simulink model "HIL_Testing_SW"  (Simulink 7.5)
settings: Solver=ode1  StartTime=0.0  StopTime=Inf  FixedStep=0.001  RelTol=1e-3
PostLoadFcn:
  | , if any(exist('dsrtsu_mdlpostloadfcn', 'file') == [2, 3, 6]), try dsrtsu_mdlpostloadfcn('Execute', bdroot); catch fprintf('Error in PostLoadFcn (dsrtsu_mdlpostloadfcn) for model "%s":\n %s\n', bdroot, lasterr); end, end,
undefined symbols (not defined in the file): CeBSER_Cnt_NumTempAxisPts, ChargeCord, ChargeCord_Control, ChargeToSOCCurr, ChrgCurrLim, CrntSens1Fine, CS_SOCSetPt, CyclerMaxChrgPwr, CyclerMaxDschrgPwr, deltaAhr, Drive_1, Drive_10, Drive_11, Drive_12, Drive_13, Drive_14, Drive_15, Drive_16, Drive_17, Drive_18, Drive_19, Drive_2, Drive_20, Drive_21, Drive_22, Drive_23, Drive_24, Drive_25, Drive_26, Drive_27, Drive_28, Drive_29, Drive_3, Drive_30, Drive_31, Drive_32, Drive_33, Drive_34, Drive_35, Drive_36, Drive_37, Drive_38, Drive_39, Drive_4, Drive_40, Drive_41, Drive_42, Drive_43, Drive_44, Drive_45, Drive_46, Drive_47, Drive_48, Drive_49, Drive_5, Drive_50, Drive_51, Drive_6, Drive_7, Drive_8 ... (+50)
libraries: simulink x129, rtican x50, rti2211sailib x5, rti2211serlib x5, rti2202miolib x3
(part 19 of 23)

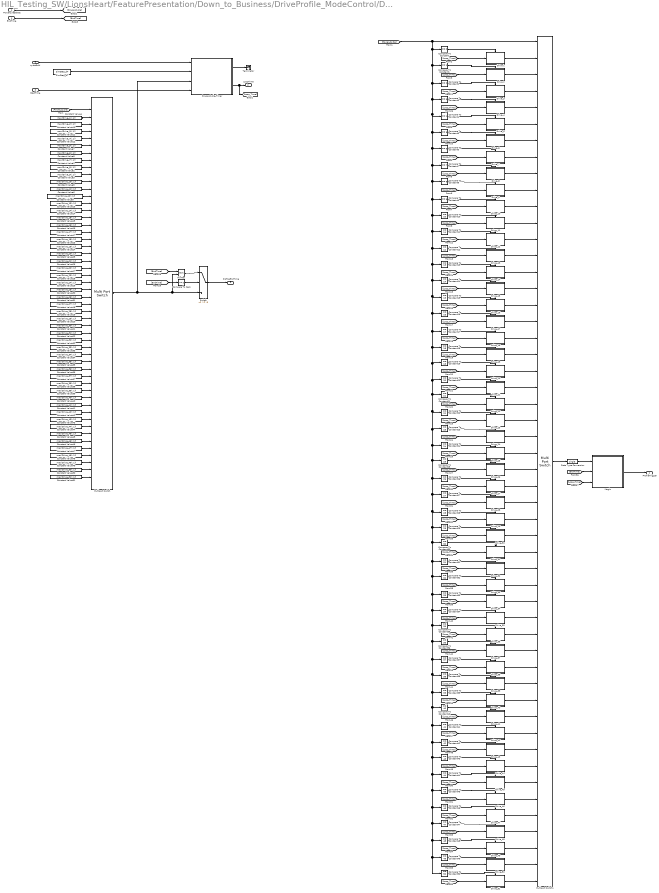
== system HIL_Testing_SW/LionsHeart/FeaturePresentation/Down_to_Business/DriveProfile_ModeControl/Drive_Profile/CD ==
  PowercyleSelect : Inport  OutDataType=fixdt(1, 16)  OutScaling=2^0
  cycleEnbl : Inport  Port=2  OutDataType=fixdt(1, 16)  OutScaling=2^0
  StartTime : Inport  Port=3  OutDataType=fixdt(1, 16)  OutScaling=2^0
  EndTime : Inport  Port=4  OutDataType=fixdt(1, 16)  OutScaling=2^0
  Compare To Constant : simulink/Logic and Bit Operations/Compare To Constant  SystemSampleTime=-1  relop===  const=0  LogicOutDataTypeMode=uint8
  Compare To Constant1 : simulink/Logic and Bit Operations/Compare To Constant  SystemSampleTime=-1  relop===  const=1  LogicOutDataTypeMode=uint8
  Compare To Constant10 : simulink/Logic and Bit Operations/Compare To Constant  SystemSampleTime=-1  relop===  const=10  LogicOutDataTypeMode=uint8
  Compare To Constant11 : simulink/Logic and Bit Operations/Compare To Constant  SystemSampleTime=-1  relop===  const=11  LogicOutDataTypeMode=uint8
  Compare To Constant12 : simulink/Logic and Bit Operations/Compare To Constant  SystemSampleTime=-1  relop===  const=12  LogicOutDataTypeMode=uint8
  Compare To Constant13 : simulink/Logic and Bit Operations/Compare To Constant  SystemSampleTime=-1  relop===  const=13  LogicOutDataTypeMode=uint8
  Compare To Constant14 : simulink/Logic and Bit Operations/Compare To Constant  SystemSampleTime=-1  relop===  const=14  LogicOutDataTypeMode=uint8
  Compare To Constant15 : simulink/Logic and Bit Operations/Compare To Constant  SystemSampleTime=-1  relop===  const=15  LogicOutDataTypeMode=uint8
  Compare To Constant16 : simulink/Logic and Bit Operations/Compare To Constant  SystemSampleTime=-1  relop===  const=16  LogicOutDataTypeMode=uint8
  Compare To Constant17 : simulink/Logic and Bit Operations/Compare To Constant  SystemSampleTime=-1  relop===  const=17  LogicOutDataTypeMode=uint8
  Compare To Constant18 : simulink/Logic and Bit Operations/Compare To Constant  SystemSampleTime=-1  relop===  const=18  LogicOutDataTypeMode=uint8
  Compare To Constant19 : simulink/Logic and Bit Operations/Compare To Constant  SystemSampleTime=-1  relop===  const=19  LogicOutDataTypeMode=uint8
  Compare To Constant2 : simulink/Logic and Bit Operations/Compare To Constant  SystemSampleTime=-1  relop===  const=2  LogicOutDataTypeMode=uint8
  Compare To Constant20 : simulink/Logic and Bit Operations/Compare To Constant  SystemSampleTime=-1  relop===  const=20  LogicOutDataTypeMode=uint8
  Compare To Constant21 : simulink/Logic and Bit Operations/Compare To Constant  SystemSampleTime=-1  relop===  const=21  LogicOutDataTypeMode=uint8
  Compare To Constant22 : simulink/Logic and Bit Operations/Compare To Constant  SystemSampleTime=-1  relop===  const=22  LogicOutDataTypeMode=uint8
  Compare To Constant23 : simulink/Logic and Bit Operations/Compare To Constant  SystemSampleTime=-1  relop===  const=23  LogicOutDataTypeMode=uint8
  Compare To Constant24 : simulink/Logic and Bit Operations/Compare To Constant  SystemSampleTime=-1  relop===  const=24  LogicOutDataTypeMode=uint8
  Compare To Constant25 : simulink/Logic and Bit Operations/Compare To Constant  SystemSampleTime=-1  relop===  const=25  LogicOutDataTypeMode=uint8
  Compare To Constant26 : simulink/Logic and Bit Operations/Compare To Constant  SystemSampleTime=-1  relop===  const=26  LogicOutDataTypeMode=uint8
  Compare To Constant27 : simulink/Logic and Bit Operations/Compare To Constant  SystemSampleTime=-1  relop===  const=27  LogicOutDataTypeMode=uint8
  Compare To Constant28 : simulink/Logic and Bit Operations/Compare To Constant  SystemSampleTime=-1  relop===  const=28  LogicOutDataTypeMode=uint8
  Compare To Constant29 : simulink/Logic and Bit Operations/Compare To Constant  SystemSampleTime=-1  relop===  const=29  LogicOutDataTypeMode=uint8
  Compare To Constant3 : simulink/Logic and Bit Operations/Compare To Constant  SystemSampleTime=-1  relop===  const=3  LogicOutDataTypeMode=uint8
  Compare To Constant30 : simulink/Logic and Bit Operations/Compare To Constant  SystemSampleTime=-1  relop===  const=30  LogicOutDataTypeMode=uint8
  Compare To Constant31 : simulink/Logic and Bit Operations/Compare To Constant  SystemSampleTime=-1  relop===  const=31  LogicOutDataTypeMode=uint8
  Compare To Constant32 : simulink/Logic and Bit Operations/Compare To Constant  SystemSampleTime=-1  relop===  const=32  LogicOutDataTypeMode=uint8
  Compare To Constant33 : simulink/Logic and Bit Operations/Compare To Constant  SystemSampleTime=-1  relop===  const=33  LogicOutDataTypeMode=uint8
  Compare To Constant34 : simulink/Logic and Bit Operations/Compare To Constant  SystemSampleTime=-1  relop===  const=34  LogicOutDataTypeMode=uint8
  Compare To Constant35 : simulink/Logic and Bit Operations/Compare To Constant  SystemSampleTime=-1  relop===  const=35  LogicOutDataTypeMode=uint8
  Compare To Constant36 : simulink/Logic and Bit Operations/Compare To Constant  SystemSampleTime=-1  relop===  const=36  LogicOutDataTypeMode=uint8
  Compare To Constant37 : simulink/Logic and Bit Operations/Compare To Constant  SystemSampleTime=-1  relop===  const=37  LogicOutDataTypeMode=uint8
  Compare To Constant38 : simulink/Logic and Bit Operations/Compare To Constant  SystemSampleTime=-1  relop===  const=38  LogicOutDataTypeMode=uint8
  Compare To Constant39 : simulink/Logic and Bit Operations/Compare To Constant  SystemSampleTime=-1  relop===  const=39  LogicOutDataTypeMode=uint8
  Compare To Constant4 : simulink/Logic and Bit Operations/Compare To Constant  SystemSampleTime=-1  relop===  const=4  LogicOutDataTypeMode=uint8
  Compare To Constant40 : simulink/Logic and Bit Operations/Compare To Constant  SystemSampleTime=-1  relop===  const=40  LogicOutDataTypeMode=uint8
  Compare To Constant41 : simulink/Logic and Bit Operations/Compare To Constant  SystemSampleTime=-1  relop===  const=41  LogicOutDataTypeMode=uint8
  Compare To Constant42 : simulink/Logic and Bit Operations/Compare To Constant  SystemSampleTime=-1  relop===  const=42  LogicOutDataTypeMode=uint8
  Compare To Constant43 : simulink/Logic and Bit Operations/Compare To Constant  SystemSampleTime=-1  relop===  const=43  LogicOutDataTypeMode=uint8
  Compare To Constant44 : simulink/Logic and Bit Operations/Compare To Constant  SystemSampleTime=-1  relop===  const=44  LogicOutDataTypeMode=uint8
  Compare To Constant45 : simulink/Logic and Bit Operations/Compare To Constant  SystemSampleTime=-1  relop===  const=45  LogicOutDataTypeMode=uint8
  Compare To Constant46 : simulink/Logic and Bit Operations/Compare To Constant  SystemSampleTime=-1  relop===  const=46  LogicOutDataTypeMode=uint8
  Compare To Constant47 : simulink/Logic and Bit Operations/Compare To Constant  SystemSampleTime=-1  relop===  const=47  LogicOutDataTypeMode=uint8
  Compare To Constant48 : simulink/Logic and Bit Operations/Compare To Constant  SystemSampleTime=-1  relop===  const=48  LogicOutDataTypeMode=uint8
  Compare To Constant49 : simulink/Logic and Bit Operations/Compare To Constant  SystemSampleTime=-1  relop===  const=49  LogicOutDataTypeMode=uint8
  Compare To Constant5 : simulink/Logic and Bit Operations/Compare To Constant  SystemSampleTime=-1  relop===  const=5  LogicOutDataTypeMode=uint8
  Compare To Constant50 : simulink/Logic and Bit Operations/Compare To Constant  SystemSampleTime=-1  relop===  const=50  LogicOutDataTypeMode=uint8
  Compare To Constant6 : simulink/Logic and Bit Operations/Compare To Constant  SystemSampleTime=-1  relop===  const=6  LogicOutDataTypeMode=uint8
  Compare To Constant7 : simulink/Logic and Bit Operations/Compare To Constant  SystemSampleTime=-1  relop===  const=7  LogicOutDataTypeMode=uint8
  Compare To Constant8 : simulink/Logic and Bit Operations/Compare To Constant  SystemSampleTime=-1  relop===  const=8  LogicOutDataTypeMode=uint8
  Compare To Constant9 : simulink/Logic and Bit Operations/Compare To Constant  SystemSampleTime=-1  relop===  const=9  LogicOutDataTypeMode=uint8
  Compare To Zero : simulink/Logic and Bit Operations/Compare To Zero  SystemSampleTime=-1  relop=~=  LogicOutDataTypeMode=boolean
  Constant Value1 : Constant  Tag=R12-1  Value=max(Drive_7(:,1))  OutDataType=sfix(16)  OutScaling=2^0
  Constant Value10 : Constant  Tag=R12-1  Value=max(Drive_2(:,1))  OutDataType=sfix(16)  OutScaling=2^0
  Constant Value11 : Constant  Tag=R12-1  Value=max(Drive_3(:,1))  OutDataType=sfix(16)  OutScaling=2^0
  Constant Value12 : Constant  Tag=R12-1  Value=max(Drive_4(:,1))  OutDataType=sfix(16)  OutScaling=2^0
  Constant Value13 : Constant  Tag=R12-1  Value=max(Drive_13(:,1))  OutDataType=sfix(16)  OutScaling=2^0
  Constant Value14 : Constant  Tag=R12-1  Value=max(Drive_14(:,1))  OutDataType=sfix(16)  OutScaling=2^0
  Constant Value15 : Constant  Tag=R12-1  Value=max(Drive_15(:,1))  OutDataType=sfix(16)  OutScaling=2^0
  Constant Value16 : Constant  Tag=R12-1  Value=max(Drive_16(:,1))  OutDataType=sfix(16)  OutScaling=2^0
  Constant Value17 : Constant  Tag=R12-1  Value=max(Drive_17(:,1))  OutDataType=sfix(16)  OutScaling=2^0
  Constant Value18 : Constant  Tag=R12-1  Value=max(Drive_27(:,1))  OutDataType=sfix(16)  OutScaling=2^0
  Constant Value19 : Constant  Tag=R12-1  Value=max(Drive_28(:,1))  OutDataType=sfix(16)  OutScaling=2^0
  Constant Value2 : Constant  Tag=R12-1  Value=max(Drive_8(:,1))  OutDataType=sfix(16)  OutScaling=2^0
  Constant Value20 : Constant  Tag=R12-1  Value=max(Drive_29(:,1))  OutDataType=sfix(16)  OutScaling=2^0
  Constant Value21 : Constant  Tag=R12-1  Value=max(Drive_30(:,1))  OutDataType=sfix(16)  OutScaling=2^0
  Constant Value22 : Constant  Tag=R12-1  Value=max(Drive_31(:,1))  OutDataType=sfix(16)  OutScaling=2^0
  Constant Value23 : Constant  Tag=R12-1  Value=max(Drive_18(:,1))  OutDataType=sfix(16)  OutScaling=2^0
  Constant Value24 : Constant  Tag=R12-1  Value=max(Drive_19(:,1))  OutDataType=sfix(16)  OutScaling=2^0
  Constant Value25 : Constant  Tag=R12-1  Value=max(Drive_20(:,1))  OutDataType=sfix(16)  OutScaling=2^0
  Constant Value26 : Constant  Tag=R12-1  Value=max(Drive_21(:,1))  OutDataType=sfix(16)  OutScaling=2^0
  Constant Value27 : Constant  Tag=R12-1  Value=max(Drive_22(:,1))  OutDataType=sfix(16)  OutScaling=2^0
  Constant Value28 : Constant  Tag=R12-1  Value=max(Drive_23(:,1))  VectorParams1D=off  OutDataType=sfix(16)  OutScaling=2^0
  Constant Value29 : Constant  Tag=R12-1  Value=max(Drive_24(:,1))  OutDataType=sfix(16)  OutScaling=2^0
  Constant Value3 : Constant  Tag=R12-1  Value=max(Drive_9(:,1))  OutDataType=sfix(16)  OutScaling=2^0
  Constant Value30 : Constant  Tag=R12-1  Value=max(Drive_25(:,1))  OutDataType=sfix(16)  OutScaling=2^0
  Constant Value31 : Constant  Tag=R12-1  Value=max(Drive_26(:,1))  OutDataType=sfix(16)  OutScaling=2^0
  Constant Value32 : Constant  Tag=R12-1  Value=max(Drive_32(:,1))  OutDataType=sfix(16)  OutScaling=2^0
  Constant Value33 : Constant  Tag=R12-1  Value=max(Drive_33(:,1))  OutDataType=sfix(16)  OutScaling=2^0
  Constant Value34 : Constant  Tag=R12-1  Value=max(Drive_34(:,1))  OutDataType=sfix(16)  OutScaling=2^0
  Constant Value35 : Constant  Tag=R12-1  Value=max(Drive_35(:,1))  OutDataType=sfix(16)  OutScaling=2^0
  Constant Value36 : Constant  Tag=R12-1  Value=max(Drive_36(:,1))  OutDataType=sfix(16)  OutScaling=2^0
  Constant Value37 : Constant  Tag=R12-1  Value=max(Drive_37(:,1))  OutDataType=sfix(16)  OutScaling=2^0
  Constant Value38 : Constant  Tag=R12-1  Value=max(Drive_38(:,1))  OutDataType=sfix(16)  OutScaling=2^0
  Constant Value39 : Constant  Tag=R12-1  Value=max(Drive_39(:,1))  OutDataType=sfix(16)  OutScaling=2^0
  Constant Value4 : Constant  Tag=R12-1  Value=max(Drive_1(:,1))  OutDataType=sfix(16)  OutScaling=2^0
  Constant Value40 : Constant  Tag=R12-1  Value=max(Drive_40(:,1))  OutDataType=sfix(16)  OutScaling=2^0
  Constant Value41 : Constant  Tag=R12-1  Value=max(Drive_41(:,1))  OutDataType=sfix(16)  OutScaling=2^0
  Constant Value42 : Constant  Tag=R12-1  Value=max(Drive_42(:,1))  OutDataType=sfix(16)  OutScaling=2^0
  Constant Value43 : Constant  Tag=R12-1  Value=max(Drive_43(:,1))  OutDataType=sfix(16)  OutScaling=2^0
  Constant Value44 : Constant  Tag=R12-1  Value=max(Drive_44(:,1))  OutDataType=sfix(16)  OutScaling=2^0
  Constant Value45 : Constant  Tag=R12-1  Value=max(Drive_45(:,1))  OutDataType=sfix(16)  OutScaling=2^0
  Constant Value46 : Constant  Tag=R12-1  Value=max(Drive_46(:,1))  OutDataType=sfix(16)  OutScaling=2^0
  Constant Value47 : Constant  Tag=R12-1  Value=max(Drive_47(:,1))  OutDataType=sfix(16)  OutScaling=2^0
  Constant Value48 : Constant  Tag=R12-1  Value=max(Drive_48(:,1))  OutDataType=sfix(16)  OutScaling=2^0
  Constant Value49 : Constant  Tag=R12-1  Value=max(Drive_49(:,1))  OutDataType=sfix(16)  OutScaling=2^0
  Constant Value5 : Constant  Tag=R12-1  Value=max(Drive_10(:,1))  OutDataType=sfix(16)  OutScaling=2^0
  Constant Value50 : Constant  Tag=R12-1  Value=max(Drive_50(:,1))  OutDataType=sfix(16)  OutScaling=2^0
  Constant Value51 : Constant  Tag=R12-1  Value=max(Drive_51(:,1))  OutDataType=sfix(16)  OutScaling=2^0
  Constant Value6 : Constant  Tag=R12-1  Value=max(Drive_11(:,1))  OutDataType=sfix(16)  OutScaling=2^0
  Constant Value7 : Constant  Tag=R12-1  Value=max(Drive_5(:,1))  OutDataType=sfix(16)  OutScaling=2^0
  Constant Value8 : Constant  Tag=R12-1  Value=max(Drive_6(:,1))  VectorParams1D=off  OutDataType=sfix(16)  OutScaling=2^0
  Constant Value9 : Constant  Tag=R12-1  Value=max(Drive_12(:,1))  OutDataType=sfix(16)  OutScaling=2^0
  Data Type Conversion : DataTypeConversion  OutDataTypeMode=single  OutDataType=sfix(16)  OutScaling=2^0  OutDataTypeStr=single
  Drive 1 : Subsystem  Tag=x.x
      mask Type: Subsystem
      mask Display:
      | text(.52,.01,char(get_param(gcb,'Tag') ), 'horizontalAlignment','center','verticalAlignment','bottom' )
      | disp(get_param(gcb,'Name'))
  Drive 2 : Subsystem  Tag=x.x
      mask Type: Subsystem
      mask Display:
      | text(.52,.01,char(get_param(gcb,'Tag') ), 'horizontalAlignment','center','verticalAlignment','bottom' )
      | disp(get_param(gcb,'Name'))
  Drive_10 : Subsystem  Tag=x.x
      mask Type: Subsystem
      mask Display:
      | text(.52,.01,char(get_param(gcb,'Tag') ), 'horizontalAlignment','center','verticalAlignment','bottom' )
      | disp(get_param(gcb,'Name'))
  Drive_11 : Subsystem  Tag=x.x
      mask Type: Subsystem
      mask Display:
      | text(.52,.01,char(get_param(gcb,'Tag') ), 'horizontalAlignment','center','verticalAlignment','bottom' )
      | disp(get_param(gcb,'Name'))
  Drive_12 : Subsystem  Tag=x.x
      mask Type: Subsystem
      mask Display:
      | text(.52,.01,char(get_param(gcb,'Tag') ), 'horizontalAlignment','center','verticalAlignment','bottom' )
      | disp(get_param(gcb,'Name'))
  Drive_13 : Subsystem  Tag=x.x
      mask Type: Subsystem
      mask Display:
      | text(.52,.01,char(get_param(gcb,'Tag') ), 'horizontalAlignment','center','verticalAlignment','bottom' )
      | disp(get_param(gcb,'Name'))
  Drive_14 : Subsystem  Tag=x.x
      mask Type: Subsystem
      mask Display:
      | text(.52,.01,char(get_param(gcb,'Tag') ), 'horizontalAlignment','center','verticalAlignment','bottom' )
      | disp(get_param(gcb,'Name'))
  Drive_15 : Subsystem  Tag=x.x
      mask Type: Subsystem
      mask Display:
      | text(.52,.01,char(get_param(gcb,'Tag') ), 'horizontalAlignment','center','verticalAlignment','bottom' )
      | disp(get_param(gcb,'Name'))
  Drive_16 : Subsystem  Tag=x.x
      mask Type: Subsystem
      mask Display:
      | text(.52,.01,char(get_param(gcb,'Tag') ), 'horizontalAlignment','center','verticalAlignment','bottom' )
      | disp(get_param(gcb,'Name'))
  Drive_17 : Subsystem  Tag=x.x
      mask Type: Subsystem
      mask Display:
      | text(.52,.01,char(get_param(gcb,'Tag') ), 'horizontalAlignment','center','verticalAlignment','bottom' )
      | disp(get_param(gcb,'Name'))
  Drive_18 : Subsystem  Tag=x.x
      mask Type: Subsystem
      mask Display:
      | text(.52,.01,char(get_param(gcb,'Tag') ), 'horizontalAlignment','center','verticalAlignment','bottom' )
      | disp(get_param(gcb,'Name'))
  Drive_19 : Subsystem  Tag=x.x
      mask Type: Subsystem
      mask Display:
      | text(.52,.01,char(get_param(gcb,'Tag') ), 'horizontalAlignment','center','verticalAlignment','bottom' )
      | disp(get_param(gcb,'Name'))
  Drive_20 : Subsystem  Tag=x.x
      mask Type: Subsystem
      mask Display:
      | text(.52,.01,char(get_param(gcb,'Tag') ), 'horizontalAlignment','center','verticalAlignment','bottom' )
      | disp(get_param(gcb,'Name'))
  Drive_21 : Subsystem  Tag=x.x
      mask Type: Subsystem
      mask Display:
      | text(.52,.01,char(get_param(gcb,'Tag') ), 'horizontalAlignment','center','verticalAlignment','bottom' )
      | disp(get_param(gcb,'Name'))
  Drive_22 : Subsystem  Tag=x.x
      mask Type: Subsystem
      mask Display:
      | text(.52,.01,char(get_param(gcb,'Tag') ), 'horizontalAlignment','center','verticalAlignment','bottom' )
      | disp(get_param(gcb,'Name'))
  Drive_23 : Subsystem  Tag=x.x
      mask Type: Subsystem
      mask Display:
      | text(.52,.01,char(get_param(gcb,'Tag') ), 'horizontalAlignment','center','verticalAlignment','bottom' )
      | disp(get_param(gcb,'Name'))
  Drive_24 : Subsystem  Tag=x.x
      mask Type: Subsystem
      mask Display:
      | text(.52,.01,char(get_param(gcb,'Tag') ), 'horizontalAlignment','center','verticalAlignment','bottom' )
      | disp(get_param(gcb,'Name'))
  Drive_25 : Subsystem  Tag=x.x
      mask Type: Subsystem
      mask Display:
      | text(.52,.01,char(get_param(gcb,'Tag') ), 'horizontalAlignment','center','verticalAlignment','bottom' )
      | disp(get_param(gcb,'Name'))
  Drive_26 : Subsystem  Tag=x.x
      mask Type: Subsystem
      mask Display:
      | text(.52,.01,char(get_param(gcb,'Tag') ), 'horizontalAlignment','center','verticalAlignment','bottom' )
      | disp(get_param(gcb,'Name'))
  Drive_27 : Subsystem  Tag=x.x
      mask Type: Subsystem
      mask Display:
      | text(.52,.01,char(get_param(gcb,'Tag') ), 'horizontalAlignment','center','verticalAlignment','bottom' )
      | disp(get_param(gcb,'Name'))
  Drive_28 : Subsystem  Tag=x.x
      mask Type: Subsystem
      mask Display:
      | text(.52,.01,char(get_param(gcb,'Tag') ), 'horizontalAlignment','center','verticalAlignment','bottom' )
      | disp(get_param(gcb,'Name'))
  Drive_29 : Subsystem  Tag=x.x
      mask Type: Subsystem
      mask Display:
      | text(.52,.01,char(get_param(gcb,'Tag') ), 'horizontalAlignment','center','verticalAlignment','bottom' )
      | disp(get_param(gcb,'Name'))
  Drive_3 : Subsystem  Tag=x.x
      mask Type: Subsystem
      mask Display:
      | text(.52,.01,char(get_param(gcb,'Tag') ), 'horizontalAlignment','center','verticalAlignment','bottom' )
      | disp(get_param(gcb,'Name'))
  Drive_30 : Subsystem  Tag=x.x
      mask Type: Subsystem
      mask Display:
      | text(.52,.01,char(get_param(gcb,'Tag') ), 'horizontalAlignment','center','verticalAlignment','bottom' )
      | disp(get_param(gcb,'Name'))
  Drive_31 : Subsystem  Tag=x.x
      mask Type: Subsystem
      mask Display:
      | text(.52,.01,char(get_param(gcb,'Tag') ), 'horizontalAlignment','center','verticalAlignment','bottom' )
      | disp(get_param(gcb,'Name'))
  Drive_32 : Subsystem  Tag=x.x
      mask Type: Subsystem
      mask Display:
      | text(.52,.01,char(get_param(gcb,'Tag') ), 'horizontalAlignment','center','verticalAlignment','bottom' )
      | disp(get_param(gcb,'Name'))
  Drive_33 : Subsystem  Tag=x.x
      mask Type: Subsystem
      mask Display:
      | text(.52,.01,char(get_param(gcb,'Tag') ), 'horizontalAlignment','center','verticalAlignment','bottom' )
      | disp(get_param(gcb,'Name'))
  Drive_34 : Subsystem  Tag=x.x
      mask Type: Subsystem
      mask Display:
      | text(.52,.01,char(get_param(gcb,'Tag') ), 'horizontalAlignment','center','verticalAlignment','bottom' )
      | disp(get_param(gcb,'Name'))
  Drive_35 : Subsystem  Tag=x.x
      mask Type: Subsystem
      mask Display:
      | text(.52,.01,char(get_param(gcb,'Tag') ), 'horizontalAlignment','center','verticalAlignment','bottom' )
      | disp(get_param(gcb,'Name'))
  Drive_36 : Subsystem  Tag=x.x
      mask Type: Subsystem
      mask Display:
      | text(.52,.01,char(get_param(gcb,'Tag') ), 'horizontalAlignment','center','verticalAlignment','bottom' )
      | disp(get_param(gcb,'Name'))
  Drive_37 : Subsystem  Tag=x.x
      mask Type: Subsystem
      mask Display:
      | text(.52,.01,char(get_param(gcb,'Tag') ), 'horizontalAlignment','center','verticalAlignment','bottom' )
      | disp(get_param(gcb,'Name'))
  Drive_38 : Subsystem  Tag=x.x
      mask Type: Subsystem
      mask Display:
      | text(.52,.01,char(get_param(gcb,'Tag') ), 'horizontalAlignment','center','verticalAlignment','bottom' )
      | disp(get_param(gcb,'Name'))
  Drive_39 : Subsystem  Tag=x.x
      mask Type: Subsystem
      mask Display:
      | text(.52,.01,char(get_param(gcb,'Tag') ), 'horizontalAlignment','center','verticalAlignment','bottom' )
      | disp(get_param(gcb,'Name'))
  Drive_4 : Subsystem  Tag=x.x
      mask Type: Subsystem
      mask Display:
      | text(.52,.01,char(get_param(gcb,'Tag') ), 'horizontalAlignment','center','verticalAlignment','bottom' )
      | disp(get_param(gcb,'Name'))
  Drive_40 : Subsystem  Tag=x.x
      mask Type: Subsystem
      mask Display:
      | text(.52,.01,char(get_param(gcb,'Tag') ), 'horizontalAlignment','center','verticalAlignment','bottom' )
      | disp(get_param(gcb,'Name'))
  Drive_41 : Subsystem  Tag=x.x
      mask Type: Subsystem
      mask Display:
      | text(.52,.01,char(get_param(gcb,'Tag') ), 'horizontalAlignment','center','verticalAlignment','bottom' )
      | disp(get_param(gcb,'Name'))
  Drive_42 : Subsystem  Tag=x.x
      mask Type: Subsystem
      mask Display:
      | text(.52,.01,char(get_param(gcb,'Tag') ), 'horizontalAlignment','center','verticalAlignment','bottom' )
      | disp(get_param(gcb,'Name'))
  Drive_43 : Subsystem  Tag=x.x
      mask Type: Subsystem
      mask Display:
      | text(.52,.01,char(get_param(gcb,'Tag') ), 'horizontalAlignment','center','verticalAlignment','bottom' )
      | disp(get_param(gcb,'Name'))
  Drive_44 : Subsystem  Tag=x.x
      mask Type: Subsystem
      mask Display:
      | text(.52,.01,char(get_param(gcb,'Tag') ), 'horizontalAlignment','center','verticalAlignment','bottom' )
      | disp(get_param(gcb,'Name'))
  Drive_45 : Subsystem  Tag=x.x
      mask Type: Subsystem
      mask Display:
      | text(.52,.01,char(get_param(gcb,'Tag') ), 'horizontalAlignment','center','verticalAlignment','bottom' )
      | disp(get_param(gcb,'Name'))
  Drive_46 : Subsystem  Tag=x.x
      mask Type: Subsystem
      mask Display:
      | text(.52,.01,char(get_param(gcb,'Tag') ), 'horizontalAlignment','center','verticalAlignment','bottom' )
      | disp(get_param(gcb,'Name'))
  Drive_47 : Subsystem  Tag=x.x
      mask Type: Subsystem
      mask Display:
      | text(.52,.01,char(get_param(gcb,'Tag') ), 'horizontalAlignment','center','verticalAlignment','bottom' )
      | disp(get_param(gcb,'Name'))
  Drive_48 : Subsystem  Tag=x.x
      mask Type: Subsystem
      mask Display:
      | text(.52,.01,char(get_param(gcb,'Tag') ), 'horizontalAlignment','center','verticalAlignment','bottom' )
      | disp(get_param(gcb,'Name'))
  Drive_49 : Subsystem  Tag=x.x
      mask Type: Subsystem
      mask Display:
      | text(.52,.01,char(get_param(gcb,'Tag') ), 'horizontalAlignment','center','verticalAlignment','bottom' )
      | disp(get_param(gcb,'Name'))
  Drive_5 : Subsystem  Tag=x.x
      mask Type: Subsystem
      mask Display:
      | text(.52,.01,char(get_param(gcb,'Tag') ), 'horizontalAlignment','center','verticalAlignment','bottom' )
      | disp(get_param(gcb,'Name'))
  Drive_50 : Subsystem  Tag=x.x
      mask Type: Subsystem
      mask Display:
      | text(.52,.01,char(get_param(gcb,'Tag') ), 'horizontalAlignment','center','verticalAlignment','bottom' )
      | disp(get_param(gcb,'Name'))
  Drive_51 : Subsystem  Tag=x.x
      mask Type: Subsystem
      mask Display:
      | text(.52,.01,char(get_param(gcb,'Tag') ), 'horizontalAlignment','center','verticalAlignment','bottom' )
      | disp(get_param(gcb,'Name'))
  Drive_6 : Subsystem  Tag=x.x
      mask Type: Subsystem
      mask Display:
      | text(.52,.01,char(get_param(gcb,'Tag') ), 'horizontalAlignment','center','verticalAlignment','bottom' )
      | disp(get_param(gcb,'Name'))
  Drive_7 : Subsystem  Tag=x.x
      mask Type: Subsystem
      mask Display:
      | text(.52,.01,char(get_param(gcb,'Tag') ), 'horizontalAlignment','center','verticalAlignment','bottom' )
      | disp(get_param(gcb,'Name'))
  Drive_8 : Subsystem  Tag=x.x
      mask Type: Subsystem
      mask Display:
      | text(.52,.01,char(get_param(gcb,'Tag') ), 'horizontalAlignment','center','verticalAlignment','bottom' )
      | disp(get_param(gcb,'Name'))
  Drive_9 : Subsystem  Tag=x.x
      mask Type: Subsystem
      mask Display:
      | text(.52,.01,char(get_param(gcb,'Tag') ), 'horizontalAlignment','center','verticalAlignment','bottom' )
      | disp(get_param(gcb,'Name'))
  Magic : Subsystem
  MinMax : MinMax  Inputs=2  OutDataType=fixdt(1, 16)  OutScaling=2^0
  Multiport Switch : MultiPortSwitch  DataPortOrder=Zero-based contiguous  Inputs=51  zeroidx=on
  Multiport Switch1 : MultiPortSwitch  DataPortOrder=Zero-based contiguous  Inputs=51  zeroidx=on
  Power_Cycle_Timer : Stateflow chart  TreatAsAtomicUnit=on
  SimStep_dT : Constant  Tag=R12-1  Value=SimStep_dT  OutDataTypeMode=double  OutDataType=sfix(16)  OutScaling=2^0  OutDataTypeStr=double
  Switch : Switch  Threshold=.5  OutDataType=fixdt(1, 16)  OutScaling=2^0
  Terminator : Terminator
  ProfileTrigger : Outport  OutDataType=fixdt(1, 16)  OutScaling=2^0
  LoopTime : Outport  Port=2  OutDataType=fixdt(1, 16)  OutScaling=2^0
  ProfileEndTime : Outport  Port=3  OutDataType=fixdt(1, 16)  OutScaling=2^0
  wires:
  [Loop_Time] -> Drive_17/1(loop_time)
  [Loop_Time] -> Drive_16/1(loop_time)
  [Loop_Time] -> Drive_15/1(loop_time)
  [Loop_Time] -> Drive_14/1(loop_time)
  [Loop_Time] -> Drive_13/1(loop_time)
  [Loop_Time] -> Drive_12/1(loop_time)
  [Loop_Time] -> Drive_11/1(loop_time)
  [Loop_Time] -> Drive_10/1(loop_time)
  [Loop_Time] -> Drive_9/1(loop_time)
  [Loop_Time] -> Drive_8/1(loop_time)
  [Loop_Time] -> Drive_7/1(loop_time)
  [Loop_Time] -> Drive_6/1(loop_time)
  [Loop_Time] -> Drive_5/1(loop_time)
  [Loop_Time] -> Drive_4/1(loop_time)
  [Loop_Time] -> Drive_3/1(loop_time)
  [Loop_Time] -> Drive 2/1(loop_time)
  Multiport Switch1/1 -> Data Type Conversion/1
  [Loop_Time] -> Drive 1/1(loop_time)
  [Power_Cycle] -> Multiport Switch1/1, Compare To Constant/1, Compare To Constant1/1, Compare To Constant2/1, Compare To Constant3/1, Compare To Constant4/1, Compare To Constant5/1, Compare To Constant6/1, Compare To Constant7/1, Compare To Constant8/1, Compare To Constant9/1, Compare To Constant10/1, Compare To Constant11/1, Compare To Constant12/1, Compare To Constant13/1, Compare To Constant14/1, Compare To Constant15/1, Compare To Constant16/1, Compare To Constant17/1, Compare To Constant18/1, Compare To Constant19/1, Compare To Constant20/1, Compare To Constant21/1, Compare To Constant22/1, Compare To Constant23/1, Compare To Constant24/1, Compare To Constant25/1, Compare To Constant26/1, Compare To Constant27/1, Compare To Constant28/1, Compare To Constant29/1, Compare To Constant30/1, Compare To Constant31/1, Compare To Constant32/1, Compare To Constant33/1, Compare To Constant34/1, Compare To Constant35/1, Compare To Constant36/1, Compare To Constant37/1, Compare To Constant38/1, Compare To Constant39/1, Compare To Constant40/1, Compare To Constant41/1, Compare To Constant42/1, Compare To Constant43/1, Compare To Constant44/1, Compare To Constant45/1, Compare To Constant46/1, Compare To Constant47/1, Compare To Constant48/1, Compare To Constant50/1, Compare To Constant49/1
  SimStep_dT/1 -> Power_Cycle_Timer/2(sim_time_step)
  Power_Cycle_Timer/2(loop_time) -> [Loop_Time], LoopTime/1
  Power_Cycle_Timer/1(loop_counter) -> Terminator/1
  [Power_Cycle] -> Multiport Switch/1
  Constant Value10/1 -> Multiport Switch/3
  Constant Value11/1 -> Multiport Switch/4
  Constant Value4/1 -> Multiport Switch/2
  Constant Value12/1 -> Multiport Switch/5
  Constant Value8/1 -> Multiport Switch/7
  Constant Value7/1 -> Multiport Switch/6
  Constant Value1/1 -> Multiport Switch/8
  Constant Value2/1 -> Multiport Switch/9
  Constant Value3/1 -> Multiport Switch/10
  Constant Value5/1 -> Multiport Switch/11
  Constant Value6/1 -> Multiport Switch/12
  Constant Value9/1 -> Multiport Switch/13
  Constant Value13/1 -> Multiport Switch/14
  Constant Value14/1 -> Multiport Switch/15
  Constant Value15/1 -> Multiport Switch/16
  Constant Value16/1 -> Multiport Switch/17
  Constant Value17/1 -> Multiport Switch/18
  cycleEnbl/1 -> Power_Cycle_Timer/1(cycle_enable)
  PowercyleSelect/1 -> [Power_Cycle]
  Constant Value23/1 -> Multiport Switch/19
  Constant Value24/1 -> Multiport Switch/20
  Constant Value25/1 -> Multiport Switch/21
  Constant Value26/1 -> Multiport Switch/22
  Constant Value27/1 -> Multiport Switch/23
  [Loop_Time] -> Drive_18/1(loop_time)
  [Loop_Time] -> Drive_19/1(loop_time)
  [Loop_Time] -> Drive_20/1(loop_time)
  [Loop_Time] -> Drive_21/1(loop_time)
  [Loop_Time] -> Drive_22/1(loop_time)
  Constant Value28/1 -> Multiport Switch/24
  Constant Value29/1 -> Multiport Switch/25
  Constant Value30/1 -> Multiport Switch/26
  Constant Value31/1 -> Multiport Switch/27
  [Loop_Time] -> Drive_26/1(loop_time)
  [Loop_Time] -> Drive_25/1(loop_time)
  [Loop_Time] -> Drive_24/1(loop_time)
  [Loop_Time] -> Drive_23/1(loop_time)
  StartTime/1 -> Power_Cycle_Timer/4(StartTime)
  Switch/1 -> ProfileEndTime/1
  EndTime/1 -> [EndTime]
  Compare To Zero/1 -> Switch/2
  MinMax/1 -> Switch/1
  [EndTime] -> MinMax/1
  [EndTime] -> Compare To Zero/1
  Constant Value18/1 -> Multiport Switch/28
  [Loop_Time] -> Drive_27/1(loop_time)
  Constant Value19/1 -> Multiport Switch/29
  Constant Value20/1 -> Multiport Switch/30
  Constant Value21/1 -> Multiport Switch/31
  Constant Value22/1 -> Multiport Switch/32
  [Loop_Time] -> Drive_28/1(loop_time)
  [Loop_Time] -> Drive_29/1(loop_time)
  [Loop_Time] -> Drive_30/1(loop_time)
  [Loop_Time] -> Drive_31/1(loop_time)
  Magic/1(ProfileData) -> ProfileTrigger/1
  Data Type Conversion/1 -> Magic/1(InputPower)
  [EndTime] -> Magic/2(EndTime)
  [Loop_Time] -> Magic/3(LoopTime)
  Multiport Switch/1 -> Switch/3, MinMax/2, Power_Cycle_Timer/3(cycle_duration)
  Constant Value32/1 -> Multiport Switch/33
  Constant Value33/1 -> Multiport Switch/34
  Constant Value34/1 -> Multiport Switch/35
  Constant Value35/1 -> Multiport Switch/36
  Constant Value36/1 -> Multiport Switch/37
  Constant Value37/1 -> Multiport Switch/38
  Constant Value38/1 -> Multiport Switch/39
  Constant Value39/1 -> Multiport Switch/40
  Constant Value40/1 -> Multiport Switch/41
  Constant Value41/1 -> Multiport Switch/42
  Constant Value42/1 -> Multiport Switch/43
  Constant Value43/1 -> Multiport Switch/44
  Constant Value44/1 -> Multiport Switch/45
  Constant Value45/1 -> Multiport Switch/46
  Constant Value46/1 -> Multiport Switch/47
  Constant Value47/1 -> Multiport Switch/48
  Constant Value48/1 -> Multiport Switch/49
  Constant Value49/1 -> Multiport Switch/50
  Constant Value50/1 -> Multiport Switch/51
  Constant Value51/1 -> Multiport Switch/52
  [Loop_Time] -> Drive_32/1(loop_time)
  [Loop_Time] -> Drive_33/1(loop_time)
  [Loop_Time] -> Drive_34/1(loop_time)
  [Loop_Time] -> Drive_35/1(loop_time)
  [Loop_Time] -> Drive_36/1(loop_time)
  [Loop_Time] -> Drive_37/1(loop_time)
  [Loop_Time] -> Drive_38/1(loop_time)
  [Loop_Time] -> Drive_39/1(loop_time)
  [Loop_Time] -> Drive_40/1(loop_time)
  [Loop_Time] -> Drive_41/1(loop_time)
  [Loop_Time] -> Drive_42/1(loop_time)
  [Loop_Time] -> Drive_43/1(loop_time)
  [Loop_Time] -> Drive_44/1(loop_time)
  [Loop_Time] -> Drive_45/1(loop_time)
  [Loop_Time] -> Drive_46/1(loop_time)
  [Loop_Time] -> Drive_47/1(loop_time)
  [Loop_Time] -> Drive_48/1(loop_time)
  [Loop_Time] -> Drive_49/1(loop_time)
  [Loop_Time] -> Drive_50/1(loop_time)
  Compare To Constant/1 -> Drive 1/Enable
  Drive 1/1(Profile_Data) -> Multiport Switch1/2
  Drive 2/1(Profile_Data) -> Multiport Switch1/3
  Drive_3/1(Profile_Data) -> Multiport Switch1/4
  Drive_4/1(Profile_Data) -> Multiport Switch1/5
  Drive_5/1(Profile_Data) -> Multiport Switch1/6
  Drive_6/1(Profile_Data) -> Multiport Switch1/7
  Drive_7/1(Profile_Data) -> Multiport Switch1/8
  Drive_8/1(Profile_Data) -> Multiport Switch1/9
  Drive_9/1(Profile_Data) -> Multiport Switch1/10
  Drive_10/1(Profile_Data) -> Multiport Switch1/11
  Drive_11/1(Profile_Data) -> Multiport Switch1/12
  Drive_12/1(Profile_Data) -> Multiport Switch1/13
  Drive_13/1(Profile_Data) -> Multiport Switch1/14
  Drive_14/1(Profile_Data) -> Multiport Switch1/15
  Drive_15/1(Profile_Data) -> Multiport Switch1/16
  Drive_16/1(Profile_Data) -> Multiport Switch1/17
  Drive_17/1(Profile_Data) -> Multiport Switch1/18
  Drive_18/1(Profile_Data) -> Multiport Switch1/19
  Drive_19/1(Profile_Data) -> Multiport Switch1/20
  Drive_20/1(Profile_Data) -> Multiport Switch1/21
  Drive_21/1(Profile_Data) -> Multiport Switch1/22
  Drive_22/1(Profile_Data) -> Multiport Switch1/23
  Drive_23/1(Profile_Data) -> Multiport Switch1/24
  Drive_24/1(Profile_Data) -> Multiport Switch1/25
  Drive_25/1(Profile_Data) -> Multiport Switch1/26
  Drive_26/1(Profile_Data) -> Multiport Switch1/27
  Drive_27/1(Profile_Data) -> Multiport Switch1/28
  Drive_28/1(Profile_Data) -> Multiport Switch1/29
  Drive_29/1(Profile_Data) -> Multiport Switch1/30
  Drive_30/1(Profile_Data) -> Multiport Switch1/31
  Drive_31/1(Profile_Data) -> Multiport Switch1/32
  Drive_32/1(Profile_Data) -> Multiport Switch1/33
  Drive_33/1(Profile_Data) -> Multiport Switch1/34
  Drive_34/1(Profile_Data) -> Multiport Switch1/35
  Drive_35/1(Profile_Data) -> Multiport Switch1/36
  Drive_36/1(Profile_Data) -> Multiport Switch1/37
  Drive_37/1(Profile_Data) -> Multiport Switch1/38
  Drive_38/1(Profile_Data) -> Multiport Switch1/39
  Drive_39/1(Profile_Data) -> Multiport Switch1/40
  Drive_40/1(Profile_Data) -> Multiport Switch1/41
  Drive_41/1(Profile_Data) -> Multiport Switch1/42
  Drive_42/1(Profile_Data) -> Multiport Switch1/43
  Drive_43/1(Profile_Data) -> Multiport Switch1/44
  Drive_44/1(Profile_Data) -> Multiport Switch1/45
  Drive_45/1(Profile_Data) -> Multiport Switch1/46
  Drive_46/1(Profile_Data) -> Multiport Switch1/47
  Drive_47/1(Profile_Data) -> Multiport Switch1/48
  Drive_48/1(Profile_Data) -> Multiport Switch1/49
  Drive_49/1(Profile_Data) -> Multiport Switch1/50
  Drive_50/1(Profile_Data) -> Multiport Switch1/51
  Drive_51/1(Profile_Data) -> Multiport Switch1/52
  [Loop_Time] -> Drive_51/1(loop_time)
  Compare To Constant1/1 -> Drive 2/Enable
  Compare To Constant2/1 -> Drive_3/Enable
  Compare To Constant3/1 -> Drive_4/Enable
  Compare To Constant4/1 -> Drive_5/Enable
  Compare To Constant5/1 -> Drive_6/Enable
  Compare To Constant50/1 -> Drive_51/Enable
  Compare To Constant49/1 -> Drive_50/Enable
  Compare To Constant48/1 -> Drive_49/Enable
  Compare To Constant47/1 -> Drive_48/Enable
  Compare To Constant46/1 -> Drive_47/Enable
  Compare To Constant45/1 -> Drive_46/Enable
  Compare To Constant44/1 -> Drive_45/Enable
  Compare To Constant39/1 -> Drive_40/Enable
  Compare To Constant40/1 -> Drive_41/Enable
  Compare To Constant41/1 -> Drive_42/Enable
  Compare To Constant42/1 -> Drive_43/Enable
  Compare To Constant43/1 -> Drive_44/Enable
  Compare To Constant38/1 -> Drive_39/Enable
  Compare To Constant37/1 -> Drive_38/Enable
  Compare To Constant36/1 -> Drive_37/Enable
  Compare To Constant25/1 -> Drive_26/Enable
  Compare To Constant26/1 -> Drive_27/Enable
  Compare To Constant27/1 -> Drive_28/Enable
  Compare To Constant28/1 -> Drive_29/Enable
  Compare To Constant29/1 -> Drive_30/Enable
  Compare To Constant30/1 -> Drive_31/Enable
  Compare To Constant31/1 -> Drive_32/Enable
  Compare To Constant34/1 -> Drive_35/Enable
  Compare To Constant35/1 -> Drive_36/Enable
  Compare To Constant21/1 -> Drive_22/Enable
  Compare To Constant22/1 -> Drive_23/Enable
  Compare To Constant23/1 -> Drive_24/Enable
  Compare To Constant24/1 -> Drive_25/Enable
  Compare To Constant13/1 -> Drive_14/Enable
  Compare To Constant14/1 -> Drive_15/Enable
  Compare To Constant15/1 -> Drive_16/Enable
  Compare To Constant16/1 -> Drive_17/Enable
  Compare To Constant17/1 -> Drive_18/Enable
  Compare To Constant18/1 -> Drive_19/Enable
  Compare To Constant19/1 -> Drive_20/Enable
  Compare To Constant20/1 -> Drive_21/Enable
  Compare To Constant11/1 -> Drive_12/Enable
  Compare To Constant12/1 -> Drive_13/Enable
  Compare To Constant10/1 -> Drive_11/Enable
  Compare To Constant9/1 -> Drive_10/Enable
  Compare To Constant8/1 -> Drive_9/Enable
  Compare To Constant6/1 -> Drive_7/Enable
  Compare To Constant7/1 -> Drive_8/Enable
  Compare To Constant32/1 -> Drive_33/Enable
  Compare To Constant33/1 -> Drive_34/Enable

== system HIL_Testing_SW/LionsHeart/Input Processing/Voltage Processing/ChargeTermVoltage/LookupChrgVoltageSetPoint_BSE/Switch Case Action Subsystem ==
  SOC : Inport  OutDataType=sfix(16)  OutScaling=2^0
  SF : Inport  Port=2  OutDataType=sfix(16)  OutScaling=2^0
  Action Port : ActionPort  ActionType=case
  Lookup Table : Lookup  InputValues=KnBSER_Pct_SocAxisInv1  Table=KnBSER_U_SOCv_Col_SAI1  OutDataType=sfix(16)  OutScaling=2^0
  Lookup Table1 : Lookup  InputValues=KnBSER_Pct_SocAxisInv2  Table=KnBSER_U_SOCv_Col_SAI2  OutDataType=sfix(16)  OutScaling=2^0
  Product : Product  OutDataType=sfix(16)  OutScaling=2^0  RndMeth=Zero
  Sum : Sum  OutDataType=sfix(16)  OutScaling=2^0  RndMeth=Zero
  Sum1 : Sum  Inputs=+-  OutDataType=sfix(16)  OutScaling=2^0  RndMeth=Zero
  Output Parameter : Outport  OutDataType=sfix(16)  OutScaling=2^0
  wires:
  Lookup Table/1 -> Sum/1, Sum1/1
  SOC/1 -> Lookup Table/1, Lookup Table1/1
  Lookup Table1/1 -> Sum1/2
  Sum1/1 -> Product/1
  Product/1 -> Sum/2
  Sum/1 -> Output Parameter/1
  SF/1 -> Product/2

== system HIL_Testing_SW/LionsHeart/Input Processing/Voltage Processing/ChargeTermVoltage/LookupChrgVoltageSetPoint_BSE/Switch Case Action Subsystem1 ==
  SOC : Inport  OutDataType=sfix(16)  OutScaling=2^0
  SF : Inport  Port=2  OutDataType=sfix(16)  OutScaling=2^0
  Action Port : ActionPort  ActionType=case
  Lookup Table1 : Lookup  InputValues=KnBSER_Pct_SocAxisInv2  Table=KnBSER_U_SOCv_Col_SAI2  OutDataType=sfix(16)  OutScaling=2^0
  Lookup Table2 : Lookup  InputValues=KnBSER_Pct_SocAxisInv3  Table=KnBSER_U_SOCv_Col_SAI3  OutDataType=sfix(16)  OutScaling=2^0
  Product : Product  OutDataType=sfix(16)  OutScaling=2^0  RndMeth=Zero
  Sum : Sum  OutDataType=sfix(16)  OutScaling=2^0  RndMeth=Zero
  Sum1 : Sum  Inputs=+-  OutDataType=sfix(16)  OutScaling=2^0  RndMeth=Zero
  Output Parameter : Outport  OutDataType=sfix(16)  OutScaling=2^0
  wires:
  SF/1 -> Product/2
  Sum/1 -> Output Parameter/1
  Product/1 -> Sum/2
  Sum1/1 -> Product/1
  Lookup Table2/1 -> Sum1/2
  SOC/1 -> Lookup Table1/1, Lookup Table2/1
  Lookup Table1/1 -> Sum/1, Sum1/1

== system HIL_Testing_SW/LionsHeart/Input Processing/Voltage Processing/ChargeTermVoltage/LookupChrgVoltageSetPoint_BSE/Switch Case Action Subsystem2 ==
  SOC : Inport  OutDataType=sfix(16)  OutScaling=2^0
  SF : Inport  Port=2  OutDataType=sfix(16)  OutScaling=2^0
  Action Port : ActionPort  ActionType=case
  Lookup Table1 : Lookup  InputValues=KnBSER_Pct_SocAxisInv4  Table=KnBSER_U_SOCv_Col_SAI4  OutDataType=sfix(16)  OutScaling=2^0
  Lookup Table2 : Lookup  InputValues=KnBSER_Pct_SocAxisInv3  Table=KnBSER_U_SOCv_Col_SAI3  OutDataType=sfix(16)  OutScaling=2^0
  Product : Product  OutDataType=sfix(16)  OutScaling=2^0  RndMeth=Zero
  Sum : Sum  OutDataType=sfix(16)  OutScaling=2^0  RndMeth=Zero
  Sum1 : Sum  Inputs=+-  OutDataType=sfix(16)  OutScaling=2^0  RndMeth=Zero
  Output Parameter : Outport  OutDataType=sfix(16)  OutScaling=2^0
  wires:
  Lookup Table2/1 -> Sum/1, Sum1/1
  SOC/1 -> Lookup Table2/1, Lookup Table1/1
  Lookup Table1/1 -> Sum1/2
  Sum1/1 -> Product/1
  Product/1 -> Sum/2
  Sum/1 -> Output Parameter/1
  SF/1 -> Product/2

== system HIL_Testing_SW/LionsHeart/Input Processing/Voltage Processing/ChargeTermVoltage/LookupChrgVoltageSetPoint_BSE/Switch Case Action Subsystem3 ==
  SOC : Inport  OutDataType=sfix(16)  OutScaling=2^0
  SF : Inport  Port=2  OutDataType=sfix(16)  OutScaling=2^0
  Action Port : ActionPort  ActionType=case
  Lookup Table1 : Lookup  InputValues=KnBSER_Pct_SocAxisInv4  Table=KnBSER_U_SOCv_Col_SAI4  OutDataType=sfix(16)  OutScaling=2^0
  Lookup Table2 : Lookup  InputValues=KnBSER_Pct_SocAxisInv5  Table=KnBSER_U_SOCv_Col_SAI5  OutDataType=sfix(16)  OutScaling=2^0
  Product : Product  OutDataType=sfix(16)  OutScaling=2^0  RndMeth=Zero
  Sum : Sum  OutDataType=sfix(16)  OutScaling=2^0  RndMeth=Zero
  Sum1 : Sum  Inputs=+-  OutDataType=sfix(16)  OutScaling=2^0  RndMeth=Zero
  Output Parameter : Outport  OutDataType=sfix(16)  OutScaling=2^0
  wires:
  SF/1 -> Product/2
  Sum/1 -> Output Parameter/1
  Product/1 -> Sum/2
  Sum1/1 -> Product/1
  Lookup Table2/1 -> Sum1/2
  SOC/1 -> Lookup Table1/1, Lookup Table2/1
  Lookup Table1/1 -> Sum/1, Sum1/1

== system HIL_Testing_SW/LionsHeart/Input Processing/Voltage Processing/ChargeTermVoltage/LookupChrgVoltageSetPoint_BSE/Switch Case Action Subsystem4 ==
  SOC : Inport  OutDataType=sfix(16)  OutScaling=2^0
  SF : Inport  Port=2  OutDataType=sfix(16)  OutScaling=2^0
  Action Port : ActionPort  ActionType=case
  Lookup Table1 : Lookup  InputValues=KnBSER_Pct_SocAxisInv6  Table=KnBSER_U_SOCv_Col_SAI6  OutDataType=sfix(16)  OutScaling=2^0
  Lookup Table2 : Lookup  InputValues=KnBSER_Pct_SocAxisInv5  Table=KnBSER_U_SOCv_Col_SAI5  OutDataType=sfix(16)  OutScaling=2^0
  Product : Product  OutDataType=sfix(16)  OutScaling=2^0  RndMeth=Zero
  Sum : Sum  OutDataType=sfix(16)  OutScaling=2^0  RndMeth=Zero
  Sum1 : Sum  Inputs=+-  OutDataType=sfix(16)  OutScaling=2^0  RndMeth=Zero
  Output Parameter : Outport  OutDataType=sfix(16)  OutScaling=2^0
  wires:
  Lookup Table2/1 -> Sum/1, Sum1/1
  SOC/1 -> Lookup Table2/1, Lookup Table1/1
  Lookup Table1/1 -> Sum1/2
  Sum1/1 -> Product/1
  Product/1 -> Sum/2
  Sum/1 -> Output Parameter/1
  SF/1 -> Product/2

== system HIL_Testing_SW/LionsHeart/Input Processing/Voltage Processing/ChargeTermVoltage/LookupChrgVoltageSetPoint_BSE/Switch Case Action Subsystem5 ==
  SOC : Inport  OutDataType=sfix(16)  OutScaling=2^0
  SF : Inport  Port=2  OutDataType=sfix(16)  OutScaling=2^0
  Action Port : ActionPort  ActionType=case
  Lookup Table1 : Lookup  InputValues=KnBSER_Pct_SocAxisInv6  Table=KnBSER_U_SOCv_Col_SAI6  OutDataType=sfix(16)  OutScaling=2^0
  Lookup Table2 : Lookup  InputValues=KnBSER_Pct_SocAxisInv7  Table=KnBSER_U_SOCv_Col_SAI7  OutDataType=sfix(16)  OutScaling=2^0
  Product : Product  OutDataType=sfix(16)  OutScaling=2^0  RndMeth=Zero
  Sum : Sum  OutDataType=sfix(16)  OutScaling=2^0  RndMeth=Zero
  Sum1 : Sum  Inputs=+-  OutDataType=sfix(16)  OutScaling=2^0  RndMeth=Zero
  Output Parameter : Outport  OutDataType=sfix(16)  OutScaling=2^0
  wires:
  SF/1 -> Product/2
  Sum/1 -> Output Parameter/1
  Product/1 -> Sum/2
  Sum1/1 -> Product/1
  Lookup Table2/1 -> Sum1/2
  SOC/1 -> Lookup Table1/1, Lookup Table2/1
  Lookup Table1/1 -> Sum/1, Sum1/1

== system HIL_Testing_SW/LionsHeart/Input Processing/Voltage Processing/ChargeTermVoltage/LookupChrgVoltageSetPoint_BSE/Switch Case Action Subsystem6 ==
  SOC : Inport  OutDataType=sfix(16)  OutScaling=2^0
  SF : Inport  Port=2  OutDataType=sfix(16)  OutScaling=2^0
  Action Port : ActionPort  ActionType=case
  Lookup Table1 : Lookup  InputValues=KnBSER_Pct_SocAxisInv8  Table=KnBSER_U_SOCv_Col_SAI8  OutDataType=sfix(16)  OutScaling=2^0
  Lookup Table2 : Lookup  InputValues=KnBSER_Pct_SocAxisInv7  Table=KnBSER_U_SOCv_Col_SAI7  OutDataType=sfix(16)  OutScaling=2^0
  Product : Product  OutDataType=sfix(16)  OutScaling=2^0  RndMeth=Zero
  Sum : Sum  OutDataType=sfix(16)  OutScaling=2^0  RndMeth=Zero
  Sum1 : Sum  Inputs=+-  OutDataType=sfix(16)  OutScaling=2^0  RndMeth=Zero
  Output Parameter : Outport  OutDataType=sfix(16)  OutScaling=2^0
  wires:
  Lookup Table2/1 -> Sum/1, Sum1/1
  SOC/1 -> Lookup Table2/1, Lookup Table1/1
  Lookup Table1/1 -> Sum1/2
  Sum1/1 -> Product/1
  Product/1 -> Sum/2
  Sum/1 -> Output Parameter/1
  SF/1 -> Product/2

== system HIL_Testing_SW/LionsHeart/Input Processing/Voltage Processing/ChargeTermVoltage/LookupChrgVoltageSetPoint_BSE/Switch Case Action Subsystem7 ==
  SOC : Inport  OutDataType=sfix(16)  OutScaling=2^0
  SF : Inport  Port=2  OutDataType=sfix(16)  OutScaling=2^0
  Action Port : ActionPort  ActionType=case
  Lookup Table1 : Lookup  InputValues=KnBSER_Pct_SocAxisInv8  Table=KnBSER_U_SOCv_Col_SAI8  OutDataType=sfix(16)  OutScaling=2^0
  Lookup Table2 : Lookup  InputValues=KnBSER_Pct_SocAxisInv9  Table=KnBSER_U_SOCv_Col_SAI9  OutDataType=sfix(16)  OutScaling=2^0
  Product : Product  OutDataType=sfix(16)  OutScaling=2^0  RndMeth=Zero
  Sum : Sum  OutDataType=sfix(16)  OutScaling=2^0  RndMeth=Zero
  Sum1 : Sum  Inputs=+-  OutDataType=sfix(16)  OutScaling=2^0  RndMeth=Zero
  Output Parameter : Outport  OutDataType=sfix(16)  OutScaling=2^0
  wires:
  SF/1 -> Product/2
  Sum/1 -> Output Parameter/1
  Product/1 -> Sum/2
  Sum1/1 -> Product/1
  Lookup Table2/1 -> Sum1/2
  SOC/1 -> Lookup Table1/1, Lookup Table2/1
  Lookup Table1/1 -> Sum/1, Sum1/1

== system HIL_Testing_SW/TX/Chiller/ChillerCmndTxDecision/ChillerRxProcessing/ReadChillerSP/RxReadChillerSP4Bytes ==
  Action Port : ActionPort  ActionType=elseif
  ASCIILUTable : Lookup  InputValues=[48,49,50,51,52,53,54,55,56,57]  Table=[0,1,2,3,4,5,6,7,8,9]  LookUpMeth=Use Input Nearest  OutDataTypeMode=single  OutDataType=fixdt(1, 16)  OutScaling=2^0  OutDataTypeStr=single  RndMeth=Nearest
  ASCIILUTable1 : Lookup  InputValues=[48,49,50,51,52,53,54,55,56,57]  Table=[0,1,2,3,4,5,6,7,8,9]  LookUpMeth=Use Input Nearest  OutDataTypeMode=single  OutDataType=fixdt(1, 16)  OutScaling=2^0  OutDataTypeStr=single  RndMeth=Nearest
  Add : Sum  Inputs=+++  OutDataType=fixdt(1, 16)  OutScaling=2^-10
  Constant : Constant  Value=43  OutDataTypeMode=uint16  OutDataType=fixdt(1, 16)  OutScaling=2^0  OutDataTypeStr=uint16
  Constant1 : Constant  Value=10  OutDataTypeMode=single  OutDataType=fixdt(1, 16)  OutScaling=2^0  OutDataTypeStr=single
  Constant2 : Constant  Value=0  OutDataTypeMode=single  OutDataType=fixdt(1, 16)  OutScaling=2^0  OutDataTypeStr=single
  Constant4 : Constant  Value=-1  OutDataTypeMode=single  OutDataType=fixdt(1, 16)  OutScaling=2^0  OutDataTypeStr=single
  Constant5 : Constant  OutDataTypeMode=single  OutDataType=fixdt(1, 16)  OutScaling=2^0  OutDataTypeStr=single
  Data Store Read1 : DataStoreRead  DataStoreName=RxChillerFIFO  SampleTime=-1
  Demux : Demux  Outputs=7
  Gain : Gain  ParameterDataType=fixdt(1, 16)  ParameterScaling=2^0  OutDataType=fixdt(1, 16)  OutScaling=2^0
  Product : Product  OutDataTypeMode=single  OutDataType=fixdt(1, 16)  OutScaling=2^0  OutDataTypeStr=single  RndMeth=Zero
  Product1 : Product  OutDataTypeMode=single  OutDataType=fixdt(1, 16)  OutScaling=2^0  OutDataTypeStr=single  RndMeth=Zero
  Relational Operator3 : RelationalOperator  Operator===  LogicOutDataTypeMode=boolean  LogicDataType=fixdt(0, 8)  OutDataTypeStr=boolean
  Switch : Switch  Threshold=1  OutDataTypeMode=single  OutDataType=fixdt(1, 16)  OutScaling=2^0  OutDataTypeStr=single
  Terminator{2..5} (4 alike) : Terminator
  RxReadChillerSetPoint : Outport  OutDataType=fixdt(1, 16)  OutScaling=2^0
  wires:
  [Sign] -> Product1/1
  Data Store Read1/1 -> Demux/1
  Demux/7 -> Terminator5/1
  Demux/6 -> Terminator4/1
  Demux/4 -> Terminator2/1
  Demux/3 -> [RxByteThree]
  Demux/2 -> [RxByteTwo]
  Demux/1 -> [RxByteOne]
  Add/1 -> Product1/2
  [TenthsNumber] -> Add/3
  [OnesNumber] -> Add/2
  [TensNumber] -> Add/1
  ASCIILUTable1/1 -> [OnesNumber]
  Product/1 -> [TensNumber]
  ASCIILUTable/1 -> Product/1
  [RxByteTwo] -> ASCIILUTable/1
  Constant1/1 -> Product/2
  Switch/1 -> [Sign]
  Constant4/1 -> Switch/3
  Constant5/1 -> Switch/1
  Relational Operator3/1 -> Switch/2
  [RxByteThree] -> ASCIILUTable1/1
  Constant/1 -> Relational Operator3/2
  [RxByteOne] -> Relational Operator3/1
  Constant2/1 -> [TenthsNumber]
  Demux/5 -> Terminator3/1
  Product1/1 -> Gain/1
  Gain/1 -> RxReadChillerSetPoint/1
